simulink model "Part4_3"  (R2022a)
settings: Solver=VariableStepAuto  StartTime=0.0  StopTime=20  RelTol=1e-3
settings Model: Creator=theod  LastModifiedBy=theod
settings DebuggingCC: UnconnectedInputMsg=warning  UnconnectedOutputMsg=warning  UnconnectedLineMsg=warning
settings RTWCC: DLArmComputeVersion=19.05

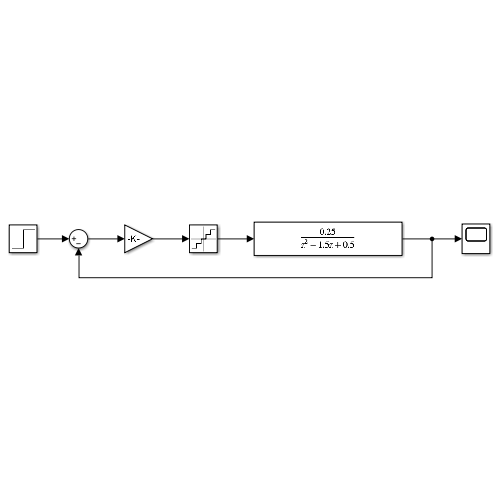
[thumbnail: Simulink's stored preview of the top-level diagram]
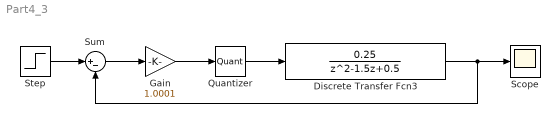
== system Part4_3 ==
  Discrete Transfer Fcn3 : DiscreteTransferFcn  Numerator=[0.25]  Denominator=[1 -1.5 0.5]
  Gain : Gain  Gain=1.0001
  Quantizer : Quantizer  QuantizationInterval=0.2
  Scope : Scope
  Step : Step  SampleTime=0.1
  Sum : Sum  Inputs=|+-
  wires:
  Sum/1 -> Gain/1
  Step/1 -> Sum/1
  Discrete Transfer Fcn3/1 -> Sum/2, Scope/1
  Quantizer/1 -> Discrete Transfer Fcn3/1
  Gain/1 -> Quantizer/1
